simulink model "Matlab_function"  (R2016a)
settings: Solver=VariableStepAuto  StartTime=0.0  StopTime=10.0  RelTol=1e-3
values from neighbouring files (symbols this model uses):
  g = 9.81    [getParams.m]    (also in sFunModell.m = block.DialogPrm(1).Data)
  l1 = 0.2    [getParams.m]    (also in sFunModell.m = block.DialogPrm(4).Data)
  l2 = 0.2    [getParams.m]    (also in sFunModell.m = block.DialogPrm(5).Data)
  m1 = 0.3    [getParams.m]    (also in sFunModell.m = block.DialogPrm(2).Data)
  m2 = 0.3    [getParams.m]    (also in sFunModell.m = block.DialogPrm(3).Data)
undefined symbols (not defined in the file or in its folder): Rp1, Rp2
settings Model: Creator=Musterstudent  LastModifiedBy=Musterstudent
settings GRTTargetCC: GeneratePreprocessorConditionals=Use local settings

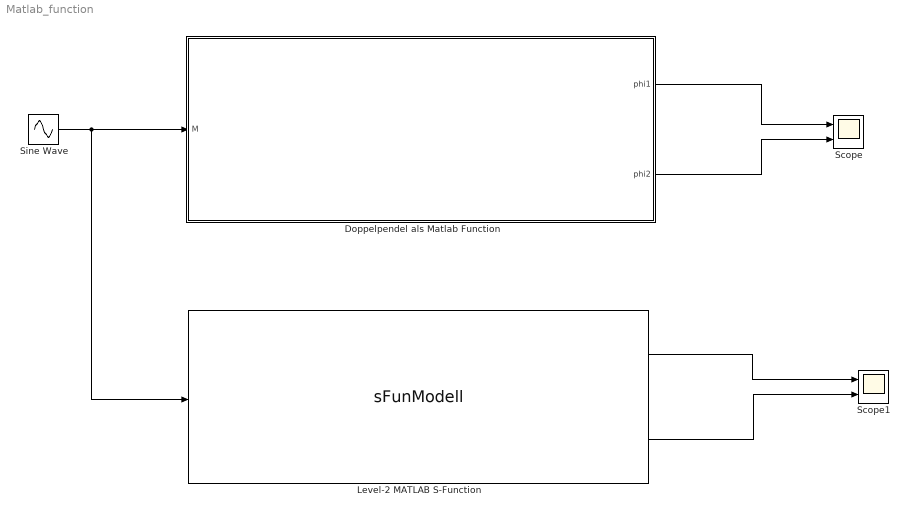
== system Matlab_function ==
  Doppelpendel als Matlab Function : Subsystem
  Level-2 MATLAB S-Function : M-S-Function  FunctionName=sFunModell  Parameters=g, m1, m2, l1, l2, Rp1, Rp2
  Scope : Scope  NumInputPorts=2
  Scope1 : Scope  NumInputPorts=2
  Sine Wave : Sin  Amplitude=0.1  SampleTime=0
  wires:
  Sine Wave/1 -> Level-2 MATLAB S-Function/1, Doppelpendel als Matlab Function/1(M)
  Doppelpendel als Matlab Function/1(phi1) -> Scope/1
  Doppelpendel als Matlab Function/2(phi2) -> Scope/2
  Level-2 MATLAB S-Function/1 -> Scope1/1
  Level-2 MATLAB S-Function/2 -> Scope1/2

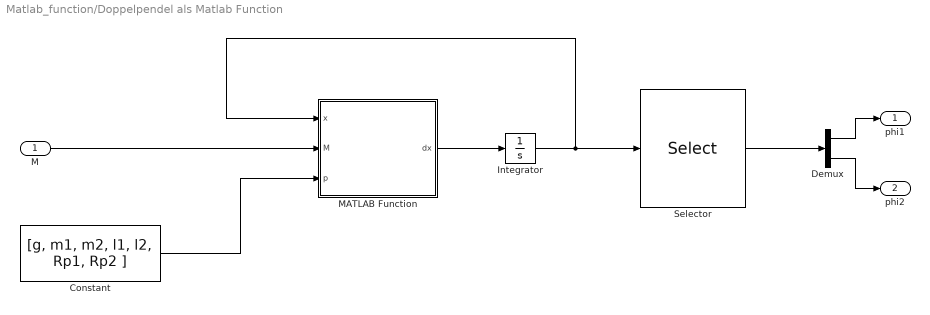
== system Matlab_function/Doppelpendel als Matlab Function ==
  M : Inport
  Constant : Constant  Value=[g, m1, m2, l1, l2, Rp1, Rp2 ]
  Demux : Demux  Outputs=2
  Integrator : Integrator  InitialCondition=[0 0 0 0]
  MATLAB Function : MATLAB Function  TreatAsAtomicUnit=on
  Selector : Selector  InputPortWidth=4  IndexOptions=Index vector (dialog)  Indices=[1 3]  OutputSizes=1
  phi1 : Outport
  phi2 : Outport  Port=2
  wires:
  M/1 -> MATLAB Function/2(M)
  Constant/1 -> MATLAB Function/3(p)
  MATLAB Function/1(dx) -> Integrator/1
  Integrator/1 -> Selector/1, MATLAB Function/1(x)
  Demux/1 -> phi1/1
  Demux/2 -> phi2/1
  Selector/1 -> Demux/1

== matlab function Matlab_function/Doppelpendel als Matlab Function/MATLAB Function ==
  data: x input; dx output; M input; p input
function dx = fcn(x,M,p)
%#codegen

phi1 = x(1);
dphi1 = x(2);
phi2 = x(3);
dphi2 = x(4);

g = p(1);
m1 = p(2);
m2 = p(3);
l1 = p(4);
l2 = p(5);
Rp1 = p(6);
Rp2 = p(7);

ddphi1 = -(24*Rp1*dphi1*l2 - 24*M*l2 + 36*Rp2*dphi1*l1*cos(phi1 - phi2) - 36*Rp2*dphi2*l1*cos(phi1 - phi2) + 9*g*l1*l2*m2*sin(phi1 - 2*phi2) + 9*dphi1^2*l1^2*l2*m2*sin(2*phi1 - 2*phi2) + 12*dphi2^2*l1*l2^2*m2*sin(phi1 - phi2) + 12*g*l1*l2*m1*sin(phi1) + 15*g*l1*l2*m2*sin(phi1))/(l1^2*l2*(8*m1 + 15*m2 - 9*m2*cos(2*phi1 - 2*phi2)));

ddphi2 = (6*(4*Rp2*dphi1*l1*m1 - 6*M*l2*m2*cos(phi1 - phi2) + 12*Rp2*dphi1*l1*m2 - 4*Rp2*dphi2*l1*m1 - 12*Rp2*dphi2*l1*m2 + 6*dphi1^2*l1^2*l2*m2^2*sin(phi1 - phi2) - 3*g*l1*l2*m2^2*sin(phi2) + (3*dphi2^2*l1*l2^2*m2^2*sin(2*phi1 - 2*phi2))/2 + 3*g*l1*l2*m2^2*sin(2*phi1 - phi2) + 6*Rp1*dphi1*l2*m2*cos(phi1 - phi2) + 2*dphi1^2*l1^2*l2*m1*m2*sin(phi1 - phi2) - (g*l1*l2*m1*m2*sin(phi2))/2 + (3*g*l1*l2*m1*m2*sin(2*phi1 - phi2))/2))/(l1*l2^2*m2*(8*m1 + 15*m2 - 9*m2*cos(2*phi1 - 2*phi2)));


dx = [dphi1, ddphi1, dphi2, ddphi2];
